simulink model "ComplexPhaseDetectorSwap"  (R2016a)
settings: Solver=VariableStepAuto  StartTime=0.0  StopTime=.05  RelTol=1e-6
PreLoadFcn:
  | Bits = 4
  | Ts=2*3/280e6
  | dBRange=11
  | maxNumErrs=500
  | maxNumBits=1e6
  | AM_Gain=AM_GainDiff;
  | AGC_Gain=AGC_GainCalc;
  | load('IIR_Coeffs.mat');
InitFcn:
  | Br= 1/(10*Ts)
  | FreqOffset=00
  | Mode=2
  | BitsPer=[2,2,1,1]
  | EbNo=50
  | N=6
undefined symbols (not defined in the file or in its folder): designMultirateFIR, DiscIntNeverNeededParam
libraries: xbsIndex_r4 x792, commfilt2 x12, commsink2 x6, dspsigops x4, commrfcorlib x2, commchan3 x2, dspfdesign x2, dspstat3 x2, dspmlti4 x1, commdigbbndpm3 x1, commrandsrc3 x1
(part 2 of 10)

== system ComplexPhaseDetectorSwap/AD9957-2 ==
  In1 : Inport
  Add3 : Sum
  Complex to Real-Imag3 : ComplexToRealImag
  FIR Interpolation : dspmlti4/FIR Interpolation  FilterSource=Auto  h=designMultirateFIR(3,1)  L=8  FilterObject=FINTERP  framing=Allow multirate processing  outputBufInitCond=0  roundingMode=Floor  overflowMode=off  firstCoeffDataTypeStr=Inherit: Same word length as input  firstCoeffMin=[]  firstCoeffMax=[]  firstCoeffLastDataTypeStr=Inherit: Same word length as input  outputDataTypeStr=Inherit: Same as accumulator  outputMin=[]  outputMax=[]  outputLastDataTypeStr=Inherit: Same as accumulator
  NCO : dspsigops/NCO  AccIncSrc=Specify via dialog  AccInc=16384*3/8  PhaseOffsetSrc=Specify via dialog  PhaseOffset=0  AccumWL=16  HasDither=off  DitherWL=4  PNgeneratorLength=19  HasPhaseQuantizer=off  TableDepth=12  HasOutputPhaseError=off  Formula=Sine and cosine  DataType=double  OutputWL=16  OutputFL=14  CompMethod=Table lookup (no interpolation)  SampleTime=Ts/8  SamplesPerFrame=1  OutputFrames=off
  PhaseDetect1 : Product
  PhaseDetect2 : Product
  Out1 : Outport
  wires:
  Add3/1 -> Out1/1
  NCO/2 -> PhaseDetect1/2
  FIR Interpolation/1 -> Complex to Real-Imag3/1
  Complex to Real-Imag3/2 -> PhaseDetect2/1
  PhaseDetect1/1 -> Add3/2
  PhaseDetect2/1 -> Add3/1
  Complex to Real-Imag3/1 -> PhaseDetect1/1
  NCO/1 -> PhaseDetect2/2
  In1/1 -> FIR Interpolation/1

== system ComplexPhaseDetectorSwap/AGCtoAWGN1 ==
  AGC : Inport
  Bias2 : Bias  Bias=100
  Gain10 : Gain  Gain=3.55
  Gain9 : Gain  Gain=-1/10
  Math Function : Math  Operator=10^u  SaturateOnIntegerOverflow=on
  Variance : Outport
  wires:
  Math Function/1 -> Gain10/1
  Gain10/1 -> Variance/1
  Gain9/1 -> Math Function/1
  Bias2/1 -> Gain9/1
  AGC/1 -> Bias2/1

== system ComplexPhaseDetectorSwap/AGCtoAWGN2 ==
  AGC : Inport
  Bias2 : Bias  Bias=100
  Gain10 : Gain  Gain=3.55
  Gain9 : Gain  Gain=-1/10
  Math Function : Math  Operator=10^u  SaturateOnIntegerOverflow=on
  Variance : Outport
  wires:
  AGC/1 -> Bias2/1
  Bias2/1 -> Gain9/1
  Gain9/1 -> Math Function/1
  Gain10/1 -> Variance/1
  Math Function/1 -> Gain10/1

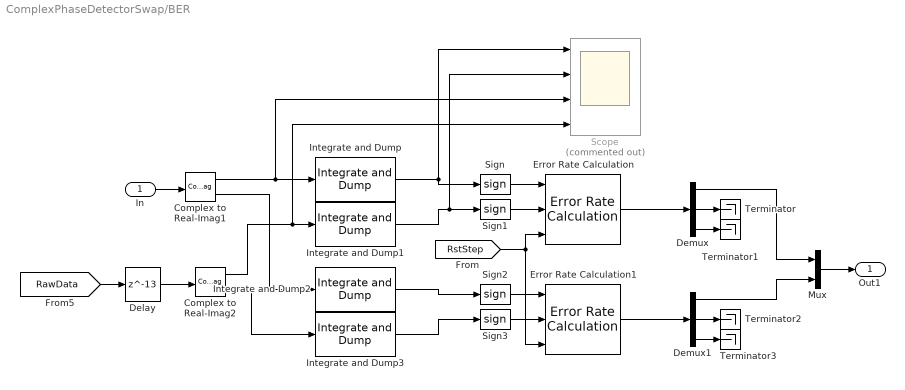
== system ComplexPhaseDetectorSwap/BER ==
  In : Inport
  Complex to Real-Imag1 : ComplexToRealImag
  Complex to Real-Imag2 : ComplexToRealImag
  Delay : Delay  DelayLength=13
  Demux : Demux  Outputs=3
  Demux1 : Demux  Outputs=3
  Error Rate Calculation : commsink2/Error Rate Calculation  N=0  st_delay=100  cp_mode=Entire frame  subframe=[]  PMode=Port  WsName=BER  RsMode2=on  stop=off  numErr=maxNumErrs  maxBits=maxNumBits
  Error Rate Calculation1 : commsink2/Error Rate Calculation  N=0  st_delay=100  cp_mode=Entire frame  subframe=[]  PMode=Port  WsName=BER  RsMode2=on  stop=off  numErr=maxNumErrs  maxBits=maxNumBits
  Integrate and Dump{,1..3} (4 alike) : commfilt2/Integrate and Dump  obssamples=1/(Br*Ts)  offsetsamples=3  nodump=off  roundingMode=Floor  overflowMode=off  outputDataTypeStr=Inherit: Same as accumulator  outputLastDataTypeStr=Inherit: Same as accumulator
  Mux : Mux  Inputs=2
  Scope : Scope  Commented=on  NumInputPorts=4
  Sign{,1..3} (4 alike) : Signum
  Terminator{,1..3} (4 alike) : Terminator
  Out1 : Outport
  wires:
  Integrate and Dump1/1 -> Scope/2, Sign1/1
  Error Rate Calculation/1 -> Demux/1
  Integrate and Dump/1 -> Scope/1, Sign/1
  Sign/1 -> Error Rate Calculation/1
  Sign1/1 -> Error Rate Calculation/2
  In/1 -> Complex to Real-Imag1/1
  Complex to Real-Imag2/1 -> Scope/4, Integrate and Dump1/1
  Delay/1 -> Complex to Real-Imag2/1
  [RawData] -> Delay/1
  Complex to Real-Imag1/1 -> Scope/3, Integrate and Dump/1
  Integrate and Dump3/1 -> Sign3/1
  Error Rate Calculation1/1 -> Demux1/1
  Integrate and Dump2/1 -> Sign2/1
  Sign2/1 -> Error Rate Calculation1/1
  Sign3/1 -> Error Rate Calculation1/2
  Complex to Real-Imag2/2 -> Integrate and Dump3/1
  [RstStep] -> Error Rate Calculation1/3, Error Rate Calculation/3
  Complex to Real-Imag1/2 -> Integrate and Dump2/1
  Demux/1 -> Mux/1
  Demux1/1 -> Mux/2
  Demux/2 -> Terminator/1
  Demux/3 -> Terminator1/1
  Demux1/2 -> Terminator2/1
  Demux1/3 -> Terminator3/1
  Mux/1 -> Out1/1

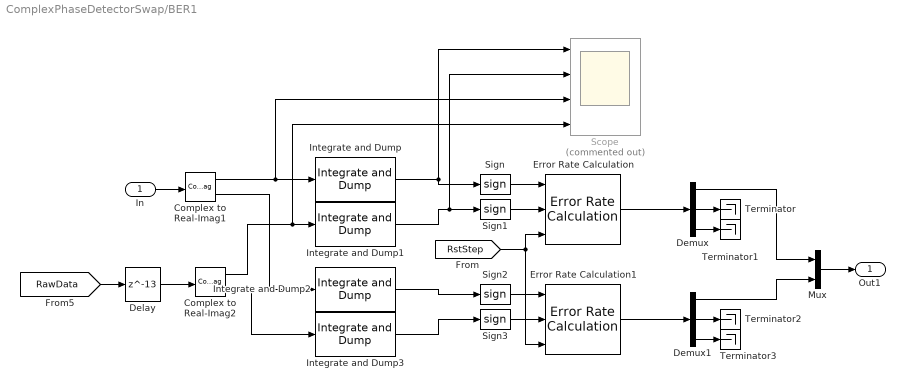
== system ComplexPhaseDetectorSwap/BER1 ==
  In : Inport
  Complex to Real-Imag1 : ComplexToRealImag
  Complex to Real-Imag2 : ComplexToRealImag
  Delay : Delay  DelayLength=13
  Demux : Demux  Outputs=3
  Demux1 : Demux  Outputs=3
  Error Rate Calculation : commsink2/Error Rate Calculation  N=0  st_delay=100  cp_mode=Entire frame  subframe=[]  PMode=Port  WsName=BER  RsMode2=on  stop=off  numErr=maxNumErrs  maxBits=maxNumBits
  Error Rate Calculation1 : commsink2/Error Rate Calculation  N=0  st_delay=100  cp_mode=Entire frame  subframe=[]  PMode=Port  WsName=BER  RsMode2=on  stop=off  numErr=maxNumErrs  maxBits=maxNumBits
  Integrate and Dump{,1..3} (4 alike) : commfilt2/Integrate and Dump  obssamples=1/(Br*Ts)  offsetsamples=3  nodump=off  roundingMode=Floor  overflowMode=off  outputDataTypeStr=Inherit: Same as accumulator  outputLastDataTypeStr=Inherit: Same as accumulator
  Mux : Mux  Inputs=2
  Scope : Scope  Commented=on  NumInputPorts=4
  Sign{,1..3} (4 alike) : Signum
  Terminator{,1..3} (4 alike) : Terminator
  Out1 : Outport
  wires:
  Mux/1 -> Out1/1
  Demux1/3 -> Terminator3/1
  Demux1/2 -> Terminator2/1
  Demux/3 -> Terminator1/1
  Demux/2 -> Terminator/1
  Demux1/1 -> Mux/2
  Demux/1 -> Mux/1
  Complex to Real-Imag1/2 -> Integrate and Dump2/1
  [RstStep] -> Error Rate Calculation/3, Error Rate Calculation1/3
  Complex to Real-Imag2/2 -> Integrate and Dump3/1
  Sign3/1 -> Error Rate Calculation1/2
  Sign2/1 -> Error Rate Calculation1/1
  Integrate and Dump2/1 -> Sign2/1
  Error Rate Calculation1/1 -> Demux1/1
  Integrate and Dump3/1 -> Sign3/1
  Complex to Real-Imag1/1 -> Integrate and Dump/1, Scope/3
  [RawData] -> Delay/1
  Delay/1 -> Complex to Real-Imag2/1
  Complex to Real-Imag2/1 -> Integrate and Dump1/1, Scope/4
  In/1 -> Complex to Real-Imag1/1
  Sign1/1 -> Error Rate Calculation/2
  Sign/1 -> Error Rate Calculation/1
  Integrate and Dump/1 -> Sign/1, Scope/1
  Error Rate Calculation/1 -> Demux/1
  Integrate and Dump1/1 -> Sign1/1, Scope/2

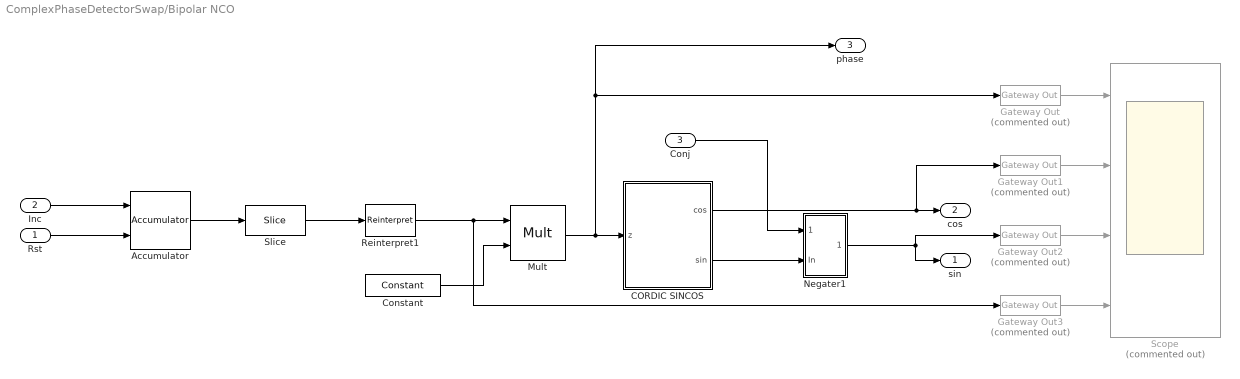
== system ComplexPhaseDetectorSwap/Bipolar NCO ==
  Rst : Inport
  Inc : Inport  Port=2
  Conj : Inport  Port=3
  Accumulator : xbsIndex_r4/Accumulator  operation=Add  n_bits=18+Bits  overflow=Wrap  scale=1  rst=on  hasbypass=off  infoeditControl=reset for floating point data type must be asserted for a minimum of 2 cycles  en=off  latency=1  msb_inp=100  msb=100  lsb=-100  use_behavioral_HDL=on  implementation=Fabric  dbl_ovrd=off  block_type=accum
  CORDIC SINCOS : Subsystem  mask(Xilinx CORDIC SINCOS){stages=17, pe_nbits=21, pe_binpt=17, pipeline_x=ones(1,17), prev_stages=17, pipeline=[1  1  1  1  1  1  1  1  1  1  1  1  1  1  1  1  1]}
      mask prompts: stages "Number of Processing Elements (integer value starting from 1)"; pe_nbits "Input Data Width"; pe_binpt "Input Binary Point Position"; pipeline_x "Latency for each Processing Element [1 0 0 1]"; prev_stages "Previous Number of Stages"; pipeline "Previous Pipeline Values"
      mask help: A parallel implementation, circular rotation mode CORDIC processor for calculating Sine and Cosine of input angle z. The number of iteration stages (and resultant output accuracy) and the processor arithmetic precision are controlled by the mask customization.
      mask init:
      | [bg,fg] = xlcmap('XBlock',0);
      | iPos = get_param(gcb,'Position');
      | iWidth=iPos(3)-iPos(1); iHeight=iPos(4)-iPos(2);
      | iCx=iWidth/2;
      | iCy=iHeight/2;
      | [logoX, logoY] = xlogo(iPos);
      | sav_gcb=gcb;
      | stages = round(sum(abs(stages)));
      | if (stages == 0)
      | 	stages = prev_stages;
      | end
      | x = zeros(1,stages);
      | pipe_size = max(size(pipeline_x));
      | if pipe_size >= stages
      | 	x(1,1:stages) = pipeline_x(1,1:stages);
      | else
      | 	x(1,1:pipe_size) = pipeline_x(1,1:pipe_size);
      | end
      | 
      | if (stages ~=prev_stages)
      | 	pipeline=x;
      | 	cordic_pe = find_system(gcb, 'lookUnderMasks', 'all', 'FollowLinks','on','masktype', 'CORDIC parallel PE');
      |     
      |   a=find_system(cordic_pe{1}, 'lookUnderMasks', 'all', 'FollowLinks','on','masktype', 'CORDIC iteration PE');
      |   for i= 2:length(a)
      |     for j=1:3
      | 	  delete_line(cordic_pe{1}, ['CORDIC PE' int2str(i-1) '/' int2str(j)], ['CORDIC PE' int2str(i) '/' int2str(j)]);
      |     end
      |   end
      |     if length(a)>0,
      |       delete_line(cordic_pe{1}, 'x/1', 'CORDIC PE1/1');
      |       delete_line(cordic_pe{1}, 'y/1', 'CORDIC PE1/2');
      |       delete_line(cordic_pe{1}, 'z/1', 'CORDIC PE1/3');
      |       delete_line(cordic_pe{1}, ['CORDIC PE' int2str(length(a)) '/1'],'X/1');
      |       delete_line(cordic_pe{1}, ['CORDIC PE' int2str(length(a)) '/2'],'Y/1');
      |       delete_line(cordic_pe{1}, ['CORDIC PE' int2str(length(a)) '/3'],'Terminator/1');
      |     elseif length(a)==0
      |       temp_port=get_param([cordic_pe{1} '/x'],'porthandles');
      |       temp_line=get_param(temp_port.Outport,'line');
      |       if temp_line>=0  delete_line(temp_line); end
      |       temp_port=get_param([cordic_pe{1} '/y'],'porthandles');
      |       temp_line=get_param(temp_port.Outport,'line');
      |       if temp_line>=0  delete_line(temp_line); end
      |       temp_port=get_param([cordic_pe{1} '/z'],'porthandles');
      |       temp_line=get_param(temp_port.Outport,'line');
      |       if temp_line>=0  delete_line(temp_line); end
      |     end
      | 
      |     for i=2:length(a)
      |       delete_block(a{i});
      |     end
      |     for i=2:stages,
      |         add_block([cordic_pe{1} '/CORDIC PE1'], [cordic_pe{1} '/CORDIC PE' int2str(i)], 'ii', int2str(i-1),'pe_nbits', 'pe_nbits','pe_binpt', 'pe_binpt','pipeline',['pipeline(1,' int2str(i) ')'],'position',[150+(i-1)*125, 70, 205+(i-1)*125, 130]);
      |     end
      | 
      |     for i= 2:stages,
      |       for j=1:3
      | 		add_line(cordic_pe{1}, ['CORDIC PE' int2str(i-1) '/' int2str(j)], ['CORDIC PE' int2str(i) '/' int2str(j)], 'autorouting', 'on');
      |       end
      |     end
      | 
      |     if stages==0
      |       add_line(cordic_pe{1}, 'x/1', 'X/1', 'autorouting', 'on');
      |       add_line(cordic_pe{1}, 'y/1', 'Terminator/1', 'autorouting', 'on');
      |       add_line(cordic_pe{1}, 'z/1', 'Z/1', 'autorouting', 'on');
      |     elseif stages>0
      |       add_line(cordic_pe{1}, 'x/1', 'CORDIC PE1/1', 'autorouting', 'on');
      |       add_line(cordic_pe{1}, 'y/1', 'CORDIC PE1/2', 'autorouting', 'on');
      |       add_line(cordic_pe{1}, 'z/1', 'CORDIC PE1/3', 'autorouting', 'on');
      | 
      |       set_param([cordic_pe{1} '/' 'X'], 'Position', [150+stages*125, 72, 180+stages*125, 86]);
      |       set_param([cordic_pe{1} '/' 'Y'], 'Position', [210+stages*125, 92, 225+stages*125, 108]);
      |       set_param([cordic_pe{1} '/' 'Terminator'], 'Position', [240+stages*125, 113, 270+stages*125, 127]);
      | 
      |       add_line(cordic_pe{1}, ['CORDIC PE' int2str(stages) '/1'], 'X/1', 'autorouting', 'on');
      |       add_line(cordic_pe{1}, ['CORDIC PE' int2str(stages) '/2'], 'Y/1', 'autorouting', 'on');
      |       add_line(cordic_pe{1}, ['CORDIC PE' int2str(stages) '/3'],'Terminator/1', 'autorouting', 'on');
      | 
      |       % force a "compile" of the constituent constant blocks to
      |       % workaround a data propagation problem
      |       find_system(cordic_pe{1}, 'lookUnderMasks', 'all', 'FollowLinks', 'on', 'MaskType','Xilinx Constant Block');
      |   end
      | 	set_param(sav_gcb, 'prev_stages', int2str(stages));
      | 	set_param(sav_gcb, 'pipeline', [ '[' int2str(x) ']']);
      | else
      | 	if (sum(pipeline~=x))
      | 		set_param(gcb, 'pipeline', [ '[' int2str(x) ']']);
      | 	end
      | end
      | str = sprintf('-%d',sum(x) + 3);
      settings: CopyFcn=set_param(gcb, 'MaskSelfModifiable', 'on', 'LinkStatus', 'none');
      mask Help: eval('');xlDoc('-book','sysgen','-topic','CORDIC_SINCOS');
      mask Display:
      | patch([0 iWidth iWidth 0],[0 0 iHeight iHeight] , bg);
      | patch(logoX,logoY , fg);
      | text(iCx-6,iCy,'z');
      | text(iCx,iCy+4,str);
      | port_label('input',1,'z');
      | port_label('output',1,'cos');
      | port_label('output',2,'sin');
      | plot([0 0 iWidth iWidth 0], [0 iHeight iHeight 0 0]);
  Constant : xbsIndex_r4/Constant  const=pi()  gui_display_data_type=Fixed-point  arith_type=Signed (2's comp)  n_bits=18  bin_pt=14  preci_type=Single  exp_width=8  frac_width=24  explicit_period=off  period=1  equ=P=C  opselect=C  inp2=PCIN>>17  opr=+  inp1=P  carry=CIN  dbl_ovrd=off  block_type=constant
  Gateway Out{,1..3} (4 alike) : xbsIndex_r4/Gateway Out  Commented=on  inherit_from_input=off  hdl_port=on  rows=1  columns=1  UseAsDAC=off  DACChannel='1'  interface=None  automatic_assignment=on  address_offset=hex2dec('00')  intf_name=''  intf_description=''  timing_constraint=None  locs_specified=off  LOCs={}  io_standard={}  block_type=gatewayout
  Mult : xbsIndex_r4/Mult  precision=User Defined  arith_type="Signed  (2's comp)"  n_bits=21  bin_pt=17  quantization=Truncate  overflow=Saturate  en=off  latency=3  use_behavioral_HDL=off  opt=Speed  use_embedded=on  optimum_pipeline=off  pipeline=on  dbl_ovrd=off  use_rpm=on  placement_style=Triangular  block_type=mult
  Negater1 : Subsystem
  Reinterpret1 : xbsIndex_r4/Reinterpret  force_arith_type=on  arith_type="Signed  (2's comp)"  force_bin_pt=on  bin_pt=17  block_type=reinterpret
  Scope : Scope  Commented=on  NumInputPorts=4
  Slice : xbsIndex_r4/Slice  nbits=18  boolean_output=off  mode=Upper Bit Location + Width  bit1=0  base1=MSB of Input  bit0=0  base0=LSB of Input  dbl_ovrd=off  block_type=slice
  sin : Outport
  cos : Outport  Port=2
  phase : Outport  Port=3
  wires:
  CORDIC SINCOS/1(cos) -> Gateway Out1/1, cos/1
  Negater1/1(Out) -> sin/1, Gateway Out2/1
  Gateway Out2/1 -> Scope/3
  Gateway Out/1 -> Scope/1
  Gateway Out1/1 -> Scope/2
  Accumulator/1 -> Slice/1
  Constant/1 -> Mult/2
  Gateway Out3/1 -> Scope/4
  Inc/1 -> Accumulator/1
  Slice/1 -> Reinterpret1/1
  Reinterpret1/1 -> Gateway Out3/1, Mult/1
  Rst/1 -> Accumulator/2
  CORDIC SINCOS/2(sin) -> Negater1/2(In)
  Conj/1 -> Negater1/1(Neg)
  Mult/1 -> phase/1, Gateway Out/1, CORDIC SINCOS/1(z)

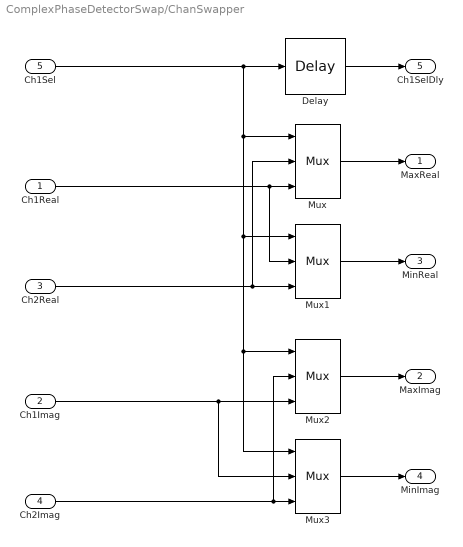
== system ComplexPhaseDetectorSwap/ChanSwapper ==
  Ch1Real : Inport
  Ch1Imag : Inport  Port=2
  Ch2Real : Inport  Port=3
  Ch2Imag : Inport  Port=4
  Ch1Sel : Inport  Port=5
  Delay : xbsIndex_r4/Delay  rst=off  infoeditControl=Selection of Reset will increase slice count due to use of real FFs and instead of SRLs  en=off  latency=1  reg_retiming=off  dbl_ovrd=off  block_type=delay
  Mux{,1..3} (4 alike) : xbsIndex_r4/Mux  inputs=2  en=off  latency=1  precision=Full  arith_type=Unsigned  n_bits=16  bin_pt=14  quantization=Truncate  overflow=Wrap  dbl_ovrd=off  block_type=mux
  MaxReal : Outport
  MaxImag : Outport  Port=2
  "MinReal " : Outport  Port=3
  MinImag : Outport  Port=4
  Ch1SelDly : Outport  Port=5
  wires:
  Ch1Sel/1 -> Mux3/1, Mux2/1, Mux1/1, Mux/1, Delay/1
  Ch2Imag/1 -> Mux2/2, Mux3/3
  Ch2Real/1 -> Mux1/3, Mux/2
  Ch1Real/1 -> Mux1/2, Mux/3
  Ch1Imag/1 -> Mux3/2, Mux2/3
  Mux/1 -> MaxReal/1
  Mux1/1 -> "MinReal "/1
  Mux2/1 -> MaxImag/1
  Mux3/1 -> MinImag/1
  Delay/1 -> Ch1SelDly/1

== system ComplexPhaseDetectorSwap/Conjugate ==
  In1 : Inport
  Complex to Real-Imag : ComplexToRealImag
  Real-Imag to Complex : RealImagToComplex
  Unary Minus : UnaryMinus
  Out1 : Outport
  wires:
  In1/1 -> Complex to Real-Imag/1
  Complex to Real-Imag/1 -> Real-Imag to Complex/1
  Complex to Real-Imag/2 -> Unary Minus/1
  Unary Minus/1 -> Real-Imag to Complex/2
  Real-Imag to Complex/1 -> Out1/1

== system ComplexPhaseDetectorSwap/Cordic ATan ==
  note: If Real=Imag=0, the Cordic goes to 180°, not 0.
  Imag : Inport
  Real : Inport  Port=2
  CORDIC ATAN : Subsystem  mask(Xilinx CORDIC ATAN){stages=10, pe_nbits=18, pe_binpt=15, pipeline_x=ones(1,10), prev_stages=10, pipeline=[1  1  1  1  1  1  1  1  1  1]}
      mask prompts: stages "Number of Processing Elements (integer value starting from 1)"; pe_nbits "X, Y Data Width"; pe_binpt "X, Y Binary Point Position"; pipeline_x "Latency for each Processing Element [1 0 0 1]"; prev_stages "Previous Number of Stages"; pipeline "Previous Pipeline Values"
      mask help: A parallel implementation, circular vectoring mode CORDIC processor for performing rectangular-to-polar conversion. The number of iteration stages (and resultant output accuracy) and the processor arithmetic precision are controlled by the mask customization.
      mask init:
      | [bg,fg] = xlcmap('XBlock',0);
      | iPos = get_param(gcb,'Position');
      | iWidth=iPos(3)-iPos(1); iHeight=iPos(4)-iPos(2);
      | iCx=iWidth/2;
      | iCy=iHeight/2;
      | [logoX, logoY] = xlogo(iPos);
      | sav_gcb=gcb;
      | stages = round(sum(abs(stages)));
      | if (stages == 0)
      | 	stages = prev_stages;
      | end
      | x = zeros(1,stages);
      | pipe_size = max(size(pipeline_x));
      | if pipe_size >= stages
      | 	x(1,1:stages) = pipeline_x(1,1:stages);
      | else
      | 	x(1,1:pipe_size) = pipeline_x(1,1:pipe_size);
      | end
      | 
      | if (stages ~=prev_stages)
      | 	pipeline=x;
      | 	cordic_pe = find_system(gcb, 'lookUnderMasks', 'all', 'FollowLinks','on','masktype', 'CORDIC parallel PE');
      |     
      |   a=find_system(cordic_pe{1}, 'lookUnderMasks', 'all', 'FollowLinks','on','masktype', 'CORDIC iteration PE');
      |   for i= 2:length(a)
      |     for j=1:3
      | 	  delete_line(cordic_pe{1}, ['CORDIC PE' int2str(i-1) '/' int2str(j)], ['CORDIC PE' int2str(i) '/' int2str(j)]);
      |     end
      |   end
      |     if length(a)>0,
      |       delete_line(cordic_pe{1}, 'x/1', 'CORDIC PE1/1');
      |       delete_line(cordic_pe{1}, 'y/1', 'CORDIC PE1/2');
      |       delete_line(cordic_pe{1}, 'z/1', 'CORDIC PE1/3');
      |       delete_line(cordic_pe{1}, ['CORDIC PE' int2str(length(a)) '/1'],'X/1');
      |       delete_line(cordic_pe{1}, ['CORDIC PE' int2str(length(a)) '/2'],'Terminator/1');
      |       delete_line(cordic_pe{1}, ['CORDIC PE' int2str(length(a)) '/3'],'Z/1');
      |     elseif length(a)==0
      |       temp_port=get_param([cordic_pe{1} '/x'],'porthandles');
      |       temp_line=get_param(temp_port.Outport,'line');
      |       if temp_line>=0  delete_line(temp_line); end
      |       temp_port=get_param([cordic_pe{1} '/y'],'porthandles');
      |       temp_line=get_param(temp_port.Outport,'line');
      |       if temp_line>=0  delete_line(temp_line); end
      |       temp_port=get_param([cordic_pe{1} '/z'],'porthandles');
      |       temp_line=get_param(temp_port.Outport,'line');
      |       if temp_line>=0  delete_line(temp_line); end
      |     end
      | 
      |     for i=2:length(a)
      |       delete_block(a{i});
      |     end
      |     for i=2:stages,
      |         add_block([cordic_pe{1} '/CORDIC PE1'], [cordic_pe{1} '/CORDIC PE' int2str(i)], 'ii', int2str(i-1),'pe_nbits', 'pe_nbits','pe_binpt', 'pe_binpt','pipeline',['pipeline(1,' int2str(i) ')'],'position',[150+(i-1)*125, 70, 205+(i-1)*125, 130]);
      |     end
      | 
      |     for i= 2:stages,
      |       for j=1:3
      | 		add_line(cordic_pe{1}, ['CORDIC PE' int2str(i-1) '/' int2str(j)], ['CORDIC PE' int2str(i) '/' int2str(j)], 'autorouting', 'on');
      |       end
      |     end
      | 
      |     if stages==0
      |       add_line(cordic_pe{1}, 'x/1', 'X/1', 'autorouting', 'on');
      |       add_line(cordic_pe{1}, 'y/1', 'Terminator/1', 'autorouting', 'on');
      |       add_line(cordic_pe{1}, 'z/1', 'Z/1', 'autorouting', 'on');
      |     elseif stages>0
      |       add_line(cordic_pe{1}, 'x/1', 'CORDIC PE1/1', 'autorouting', 'on');
      |       add_line(cordic_pe{1}, 'y/1', 'CORDIC PE1/2', 'autorouting', 'on');
      |       add_line(cordic_pe{1}, 'z/1', 'CORDIC PE1/3', 'autorouting', 'on');
      | 
      |       set_param([cordic_pe{1} '/' 'X'], 'Position', [150+stages*125, 72, 180+stages*125, 86]);
      |       set_param([cordic_pe{1} '/' 'Terminator'], 'Position', [210+stages*125, 92, 225+stages*125, 108]);
      |       set_param([cordic_pe{1} '/' 'Z'], 'Position', [240+stages*125, 113, 270+stages*125, 127]);
      | 
      |       add_line(cordic_pe{1}, ['CORDIC PE' int2str(stages) '/1'], 'X/1', 'autorouting', 'on');
      |       add_line(cordic_pe{1}, ['CORDIC PE' int2str(stages) '/2'], 'Terminator/1', 'autorouting', 'on');
      |       add_line(cordic_pe{1}, ['CORDIC PE' int2str(stages) '/3'],'Z/1', 'autorouting', 'on');
      | 
      |       % force a "compile" of the constituent constant blocks to
      |       % workaround a data propagation problem
      |       find_system(cordic_pe{1}, 'lookUnderMasks', 'all', 'FollowLinks', 'on', 'MaskType','Xilinx Constant Block');
      |   end
      | 	set_param(sav_gcb, 'prev_stages', int2str(stages));
      | 	set_param(sav_gcb, 'pipeline', [ '[' int2str(x) ']']);
      | else
      | 	if (sum(pipeline~=x))
      | 		set_param(gcb, 'pipeline', [ '[' int2str(x) ']']);
      | 	end
      | end
      | str = sprintf('-%d',sum(x) + 3);
      settings: CopyFcn=set_param(gcb, 'MaskSelfModifiable', 'on', 'LinkStatus', 'none');
      mask Help: eval('');xlDoc('-book','sysgen','-topic','CORDIC_ATAN');
      mask Display:
      | patch([0 iWidth iWidth 0],[0 0 iHeight iHeight] , bg);
      | patch(logoX,logoY , fg);
      | text(iCx-6,iCy,'z');
      | text(iCx,iCy+4,str);
      | port_label('input',1,'x');
      | port_label('input',2,'y');
      | port_label('output',1,'mag');
      | port_label('output',2,'atan');
      | plot([0 0 iWidth iWidth 0], [0 iHeight iHeight 0 0]);
  Constant : xbsIndex_r4/Constant  const=0  gui_display_data_type=Fixed-point  arith_type=Signed (2's comp)  n_bits=18  bin_pt=15  preci_type=Single  exp_width=8  frac_width=24  explicit_period=off  period=1  equ=P=C  opselect=C  inp2=PCIN>>17  opr=+  inp1=P  carry=CIN  dbl_ovrd=off  block_type=constant
  Mux : xbsIndex_r4/Mux  inputs=2  en=off  latency=1  precision=Full  arith_type=Unsigned  n_bits=16  bin_pt=14  quantization=Truncate  overflow=Wrap  dbl_ovrd=off  block_type=mux
  Relational1 : xbsIndex_r4/Relational  mode=a>b  op_type=Bool  en=off  latency=0  dbl_ovrd=off  block_type=relational
  Phase : Outport
  wires:
  Real/1 -> CORDIC ATAN/1(x)
  Imag/1 -> CORDIC ATAN/2(y)
  CORDIC ATAN/1(X) -> Relational1/1
  Mux/1 -> Phase/1
  CORDIC ATAN/2(Z) -> Mux/3
  Constant/1 -> Mux/2, Relational1/2
  Relational1/1 -> Mux/1

== system ComplexPhaseDetectorSwap/Knob ==

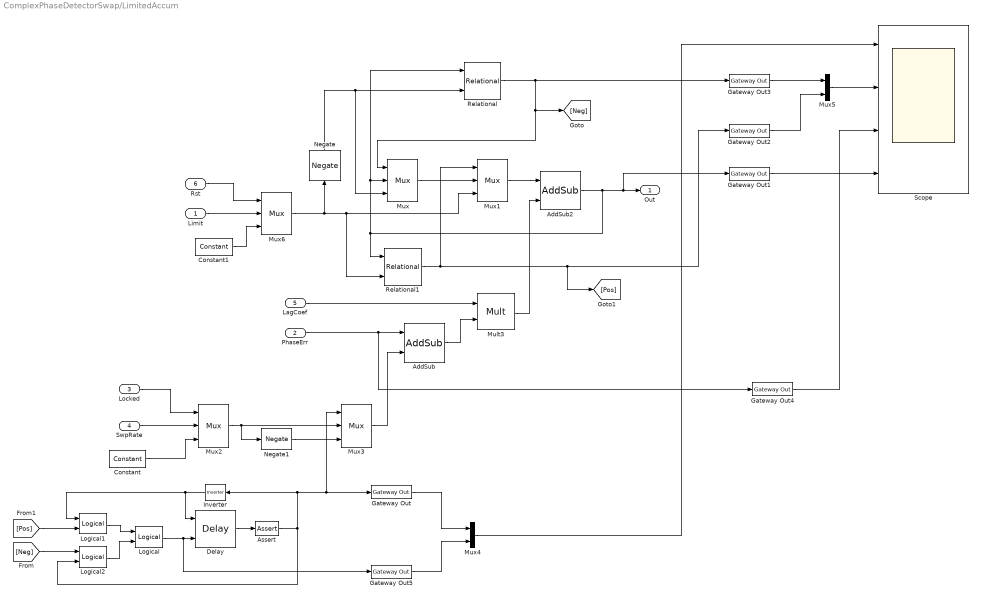
== system ComplexPhaseDetectorSwap/LimitedAccum ==
  Limit : Inport
  PhaseErr : Inport  Port=2
  Locked : Inport  Port=3
  SwpRate : Inport  Port=4
  LagCoef : Inport  Port=5
  Rst : Inport  Port=6
  AddSub : xbsIndex_r4/AddSub  mode=Addition  use_carryin=off  use_carryout=off  en=off  latency=1  precision=Full  arith_type=Unsigned  n_bits=16  bin_pt=14  quantization=Truncate  overflow=Wrap  use_behavioral_HDL=off  hw_selection=Fabric  pipelined=off  dbl_ovrd=off  block_type=addsub
  AddSub2 : xbsIndex_r4/AddSub  mode=Addition  use_carryin=off  use_carryout=off  en=off  latency=1  precision=User Defined  arith_type="Signed  (2's comp)"  n_bits=32  bin_pt=17  quantization="Round  (unbiased: +/- Inf)"  overflow=Wrap  use_behavioral_HDL=off  hw_selection=Fabric  pipelined=off  dbl_ovrd=off  block_type=addsub
  Assert : xbsIndex_r4/Assert  assert_type=on  type_source=Explicitly  gui_display_data_type=Boolean  arith_type=Boolean  n_bits=1  bin_pt=14  preci_type=Single  exp_width=8  frac_width=24  assert_rate=off  rate_source=Explicitly  period=1  output_port=on  block_type=assert
  Constant : xbsIndex_r4/Constant  const=0  gui_display_data_type=Fixed-point  arith_type=Unsigned  n_bits=8  bin_pt=5  preci_type=Single  exp_width=8  frac_width=24  explicit_period=on  period=Ts  equ=P=C  opselect=C  inp2=PCIN>>17  opr=+  inp1=P  carry=CIN  dbl_ovrd=off  block_type=constant
  Constant1 : xbsIndex_r4/Constant  const=0  gui_display_data_type=Fixed-point  arith_type=Unsigned  n_bits=14  bin_pt=0  preci_type=Single  exp_width=8  frac_width=24  explicit_period=on  period=Ts  equ=P=C  opselect=C  inp2=PCIN>>17  opr=+  inp1=P  carry=CIN  dbl_ovrd=off  block_type=constant
  Delay : xbsIndex_r4/Delay  rst=off  infoeditControl=Selection of Reset will increase slice count due to use of real FFs and instead of SRLs  en=on  latency=1  reg_retiming=off  dbl_ovrd=off  block_type=delay
  Gateway Out{,1..5} (6 alike) : xbsIndex_r4/Gateway Out  inherit_from_input=off  hdl_port=off  rows=1  columns=1  UseAsDAC=off  DACChannel='1'  interface=None  automatic_assignment=on  address_offset=hex2dec('00')  intf_name=''  intf_description=''  timing_constraint=None  locs_specified=off  LOCs={}  io_standard={}  block_type=gatewayout
  Inverter : xbsIndex_r4/Inverter  en=off  latency=0  dbl_ovrd=off  block_type=inv
  Logical : xbsIndex_r4/Logical  logical_function=OR  inputs=2  en=off  latency=0  precision=Full  arith_type=Unsigned  n_bits=16  bin_pt=0  align_bp=on  dbl_ovrd=off  block_type=logical
  Logical1 : xbsIndex_r4/Logical  logical_function=AND  inputs=2  en=off  latency=0  precision=Full  arith_type=Unsigned  n_bits=16  bin_pt=0  align_bp=on  dbl_ovrd=off  block_type=logical
  Logical2 : xbsIndex_r4/Logical  logical_function=AND  inputs=2  en=off  latency=0  precision=Full  arith_type=Unsigned  n_bits=16  bin_pt=0  align_bp=on  dbl_ovrd=off  block_type=logical
  Mult3 : xbsIndex_r4/Mult  precision=User Defined  arith_type="Signed  (2's comp)"  n_bits=18+Bits  bin_pt=17  quantization="Round  (unbiased: +/- Inf)"  overflow=Wrap  en=off  latency=3  use_behavioral_HDL=off  opt=Speed  use_embedded=on  optimum_pipeline=off  pipeline=on  dbl_ovrd=off  use_rpm=on  placement_style=Triangular  block_type=mult
  Mux{,1..2,6} (4 alike) : xbsIndex_r4/Mux  inputs=2  en=off  latency=0  precision=Full  arith_type=Unsigned  n_bits=16  bin_pt=14  quantization=Truncate  overflow=Wrap  dbl_ovrd=off  block_type=mux
  Mux3 : xbsIndex_r4/Mux  inputs=2  en=off  latency=1  precision=Full  arith_type=Unsigned  n_bits=16  bin_pt=14  quantization=Truncate  overflow=Wrap  dbl_ovrd=off  block_type=mux
  Mux4 : Mux  Inputs=2
  Mux5 : Mux  Inputs=2
  Negate : xbsIndex_r4/Negate  precision=Full  arith_type=Unsigned  n_bits=Bits+18  bin_pt=14  quantization=Truncate  overflow=Wrap  en=off  latency=0  dbl_ovrd=off  block_type=negate
  Negate1 : xbsIndex_r4/Negate  precision=Full  arith_type=Unsigned  n_bits=Bits+18  bin_pt=14  quantization=Truncate  overflow=Wrap  en=off  latency=0  dbl_ovrd=off  block_type=negate
  Relational : xbsIndex_r4/Relational  mode=a<b  op_type=Bool  en=off  latency=0  dbl_ovrd=off  block_type=relational
  Relational1 : xbsIndex_r4/Relational  mode=a>b  op_type=Bool  en=off  latency=0  dbl_ovrd=off  block_type=relational
  Scope : Scope  NumInputPorts=4
  Out : Outport
  wires:
  Mult3/1 -> AddSub2/2
  AddSub2/1 -> Relational/1, Mux/2, Relational1/1, Out/1, Gateway Out1/1
  Mux/1 -> Mux1/2
  Mux6/1 -> Negate/1, Mux1/3, Relational1/2
  Relational/1 -> [Neg], Mux/1, Gateway Out3/1
  Relational1/1 -> Mux1/1, [Pos], Gateway Out2/1
  Gateway Out1/1 -> Scope/4
  Gateway Out3/1 -> Mux5/1
  Mux4/1 -> Scope/1
  Gateway Out2/1 -> Mux5/2
  Mux1/1 -> AddSub2/1
  Negate/1 -> Relational/2, Mux/3
  PhaseErr/1 -> Gateway Out4/1, AddSub/1
  LagCoef/1 -> Mult3/1
  AddSub/1 -> Mult3/2
  Locked/1 -> Mux2/1
  Constant/1 -> Mux2/3
  Mux2/1 -> Negate1/1, Mux3/2
  SwpRate/1 -> Mux2/2
  Negate1/1 -> Mux3/3
  Mux3/1 -> AddSub/2
  Delay/1 -> Assert/1
  [Pos] -> Logical1/2
  [Neg] -> Logical2/1
  Logical/1 -> Gateway Out5/1, Delay/2
  Inverter/1 -> Delay/1, Logical1/1
  Assert/1 -> Logical2/2, Gateway Out/1, Mux3/1, Inverter/1
  Logical1/1 -> Logical/1
  Logical2/1 -> Logical/2
  Mux5/1 -> Scope/2
  Gateway Out4/1 -> Scope/3
  Gateway Out/1 -> Mux4/1
  Gateway Out5/1 -> Mux4/2
  Limit/1 -> Mux6/2
  Rst/1 -> Mux6/1
  Constant1/1 -> Mux6/3

== system ComplexPhaseDetectorSwap/LockImag ==
  In : Inport
  Sub : Inport  Port=2
  Rst_n : Inport  Port=3
  Constant : xbsIndex_r4/Constant  const=0  gui_display_data_type=Fixed-point  arith_type=Unsigned  n_bits=13  bin_pt=0  preci_type=Single  exp_width=8  frac_width=24  explicit_period=off  period=1  equ=P=C  opselect=C  inp2=PCIN>>17  opr=+  inp1=P  carry=CIN  dbl_ovrd=off  block_type=constant
  LockReal : xbsIndex_r4/AddSub  mode=Addition or Subtraction  use_carryin=off  use_carryout=off  en=off  latency=1  precision=User Defined  arith_type=Unsigned  n_bits=13  bin_pt=0  quantization=Truncate  overflow=Saturate  use_behavioral_HDL=off  hw_selection=Fabric  pipelined=off  dbl_ovrd=off  block_type=addsub
  Mux : xbsIndex_r4/Mux  inputs=2  en=off  latency=0  precision=Full  arith_type=Unsigned  n_bits=16  bin_pt=14  quantization=Truncate  overflow=Wrap  dbl_ovrd=off  block_type=mux
  Out : Outport
  wires:
  Rst_n/1 -> Mux/1
  Constant/1 -> Mux/2
  Mux/1 -> LockReal/1
  LockReal/1 -> Out/1, Mux/3
  Sub/1 -> LockReal/3
  In/1 -> LockReal/2

== system ComplexPhaseDetectorSwap/LockReal ==
  In : Inport
  Sub : Inport  Port=2
  Rst_n : Inport  Port=3
  Constant : xbsIndex_r4/Constant  const=0  gui_display_data_type=Fixed-point  arith_type=Unsigned  n_bits=13  bin_pt=0  preci_type=Single  exp_width=8  frac_width=24  explicit_period=off  period=1  equ=P=C  opselect=C  inp2=PCIN>>17  opr=+  inp1=P  carry=CIN  dbl_ovrd=off  block_type=constant
  LockReal : xbsIndex_r4/AddSub  mode=Addition or Subtraction  use_carryin=off  use_carryout=off  en=off  latency=1  precision=User Defined  arith_type=Unsigned  n_bits=13  bin_pt=0  quantization=Truncate  overflow=Saturate  use_behavioral_HDL=off  hw_selection=Fabric  pipelined=off  dbl_ovrd=off  block_type=addsub
  Mux : xbsIndex_r4/Mux  inputs=2  en=off  latency=0  precision=Full  arith_type=Unsigned  n_bits=16  bin_pt=14  quantization=Truncate  overflow=Wrap  dbl_ovrd=off  block_type=mux
  Out : Outport
  wires:
  In/1 -> LockReal/2
  Sub/1 -> LockReal/3
  LockReal/1 -> Mux/3, Out/1
  Mux/1 -> LockReal/1
  Constant/1 -> Mux/2
  Rst_n/1 -> Mux/1

== system ComplexPhaseDetectorSwap/Negater2 ==
  Neg : Inport
  In : Inport  Port=2
  Mux11 : xbsIndex_r4/Mux  inputs=2  en=off  latency=1  precision=Full  arith_type=Unsigned  n_bits=16  bin_pt=14  quantization=Truncate  overflow=Wrap  dbl_ovrd=off  block_type=mux
  Negate1 : xbsIndex_r4/Negate  precision=User Defined  arith_type="Signed  (2's comp)"  n_bits=18  bin_pt=15  quantization=Truncate  overflow=Saturate  en=off  latency=0  dbl_ovrd=off  block_type=negate
  Out : Outport
  wires:
  Neg/1 -> Mux11/1
  In/1 -> Negate1/1, Mux11/2
  Mux11/1 -> Out/1
  Negate1/1 -> Mux11/3

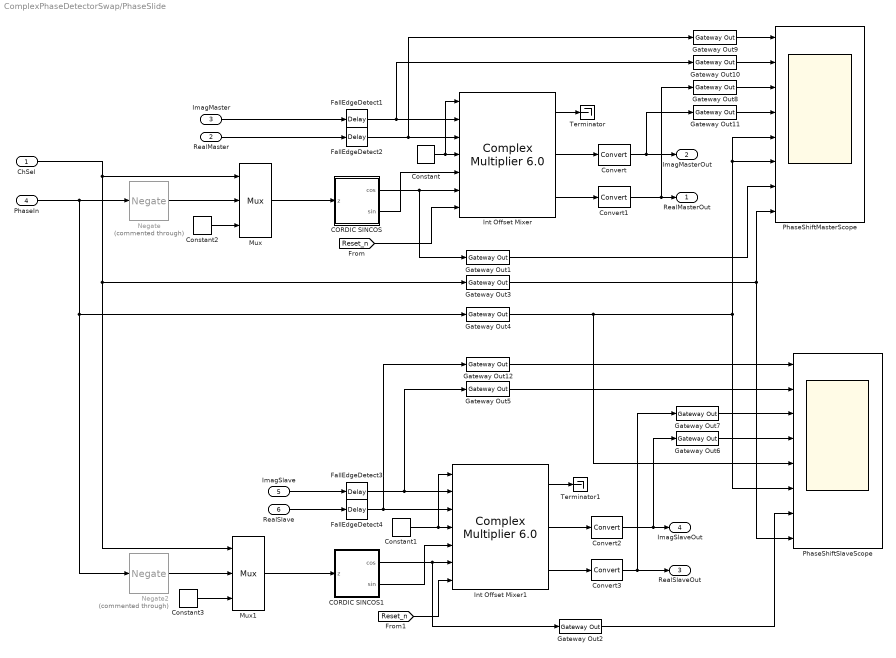
== system ComplexPhaseDetectorSwap/PhaseSlide ==
  ChSel : Inport
  RealMaster : Inport  Port=2
  ImagMaster : Inport  Port=3
  PhaseIn : Inport  Port=4
  ImagSlave : Inport  Port=5
  RealSlave : Inport  Port=6
  CORDIC SINCOS : Subsystem  mask(Xilinx CORDIC SINCOS){stages=17, pe_nbits=21, pe_binpt=17, pipeline_x=ones(1,17), prev_stages=17, pipeline=[1  1  1  1  1  1  1  1  1  1  1  1  1  1  1  1  1]}
      mask prompts: stages "Number of Processing Elements (integer value starting from 1)"; pe_nbits "Input Data Width"; pe_binpt "Input Binary Point Position"; pipeline_x "Latency for each Processing Element [1 0 0 1]"; prev_stages "Previous Number of Stages"; pipeline "Previous Pipeline Values"
      mask help: A parallel implementation, circular rotation mode CORDIC processor for calculating Sine and Cosine of input angle z. The number of iteration stages (and resultant output accuracy) and the processor arithmetic precision are controlled by the mask customization.
      mask init: same as ComplexPhaseDetectorSwap/Bipolar NCO/CORDIC SINCOS
      settings: CopyFcn=set_param(gcb, 'MaskSelfModifiable', 'on', 'LinkStatus', 'none');
      mask Help: eval('');xlDoc('-book','sysgen','-topic','CORDIC_SINCOS');
      mask Display:
      | patch([0 iWidth iWidth 0],[0 0 iHeight iHeight] , bg);
      | patch(logoX,logoY , fg);
      | text(iCx-6,iCy,'z');
      | text(iCx,iCy+4,str);
      | port_label('input',1,'z');
      | port_label('output',1,'cos');
      | port_label('output',2,'sin');
      | plot([0 0 iWidth iWidth 0], [0 iHeight iHeight 0 0]);
  CORDIC SINCOS1 : Subsystem  mask(Xilinx CORDIC SINCOS){stages=17, pe_nbits=21, pe_binpt=17, pipeline_x=ones(1,17), prev_stages=17, pipeline=[1  1  1  1  1  1  1  1  1  1  1  1  1  1  1  1  1]}
      mask prompts: stages "Number of Processing Elements (integer value starting from 1)"; pe_nbits "Input Data Width"; pe_binpt "Input Binary Point Position"; pipeline_x "Latency for each Processing Element [1 0 0 1]"; prev_stages "Previous Number of Stages"; pipeline "Previous Pipeline Values"
      mask help: A parallel implementation, circular rotation mode CORDIC processor for calculating Sine and Cosine of input angle z. The number of iteration stages (and resultant output accuracy) and the processor arithmetic precision are controlled by the mask customization.
      mask init: same as ComplexPhaseDetectorSwap/Bipolar NCO/CORDIC SINCOS
      settings: CopyFcn=set_param(gcb, 'MaskSelfModifiable', 'on', 'LinkStatus', 'none');
      mask Help: eval('');xlDoc('-book','sysgen','-topic','CORDIC_SINCOS');
      mask Display:
      | patch([0 iWidth iWidth 0],[0 0 iHeight iHeight] , bg);
      | patch(logoX,logoY , fg);
      | text(iCx-6,iCy,'z');
      | text(iCx,iCy+4,str);
      | port_label('input',1,'z');
      | port_label('output',1,'cos');
      | port_label('output',2,'sin');
      | plot([0 0 iWidth iWidth 0], [0 iHeight iHeight 0 0]);
  Constant : xbsIndex_r4/Constant  const=1  gui_display_data_type=Boolean  arith_type=Boolean  n_bits=16  bin_pt=14  preci_type=Single  exp_width=8  frac_width=24  explicit_period=on  period=Ts  equ=P=C  opselect=C  inp2=PCIN>>17  opr=+  inp1=P  carry=CIN  dbl_ovrd=off  block_type=constant
  Constant1 : xbsIndex_r4/Constant  const=1  gui_display_data_type=Boolean  arith_type=Boolean  n_bits=16  bin_pt=14  preci_type=Single  exp_width=8  frac_width=24  explicit_period=on  period=Ts  equ=P=C  opselect=C  inp2=PCIN>>17  opr=+  inp1=P  carry=CIN  dbl_ovrd=off  block_type=constant
  Constant2 : xbsIndex_r4/Constant  const=0  gui_display_data_type=Fixed-point  arith_type=Signed (2's comp)  n_bits=16  bin_pt=14  preci_type=Single  exp_width=8  frac_width=24  explicit_period=on  period=Ts  equ=P=C  opselect=C  inp2=PCIN>>17  opr=+  inp1=P  carry=CIN  dbl_ovrd=off  block_type=constant
  Constant3 : xbsIndex_r4/Constant  const=0  gui_display_data_type=Fixed-point  arith_type=Signed (2's comp)  n_bits=16  bin_pt=14  preci_type=Single  exp_width=8  frac_width=24  explicit_period=on  period=Ts  equ=P=C  opselect=C  inp2=PCIN>>17  opr=+  inp1=P  carry=CIN  dbl_ovrd=off  block_type=constant
  Convert{,1..3} (4 alike) : xbsIndex_r4/Convert  gui_display_data_type=Fixed-point  arith_type="Signed  (2's comp)"  n_bits=18  bin_pt=17  float_type=Single  exp_bits=8  fraction_bits=24  quantization=Truncate  overflow=Saturate  en=off  latency=1  pipeline=off  dbl_ovrd=off  block_type=convert
  FallEdgeDetect{1..4} (4 alike) : xbsIndex_r4/Delay  rst=off  infoeditControl=Selection of Reset will increase slice count due to use of real FFs and instead of SRLs  en=off  latency=42  reg_retiming=off  dbl_ovrd=off  block_type=delay
  Gateway Out{1..12} (12 alike) : xbsIndex_r4/Gateway Out  inherit_from_input=off  hdl_port=off  rows=1  columns=1  UseAsDAC=off  DACChannel='1'  interface=None  automatic_assignment=on  address_offset=hex2dec('00')  intf_name=''  intf_description=''  timing_constraint=None  locs_specified=off  LOCs={}  io_standard={}  block_type=gatewayout
  Int Offset Mixer : xbsIndex_r4/Complex Multiplier 6.0   hasatlast=off  hasatuser=off  atuserwidth=1  hasbtlast=off  hasbtuser=off  btuserwidth=1  multtype=Use_Mults  optimizegoal=Resources  flowcontrol=NonBlocking  outputwidth=20  roundmode=Truncate  hasctrltlast=off  hasctrltuser=off  ctrltuserwidth=1  outtlastbehv=Null  latencyconfig=Manual  minimumlatency=3  aclken=off  aresetn=on  trim_axipin_name=on  simulation_type=hybrid_sim  simulation_model=sysgen:cmpy_v6_0  data_path_portlist={ 's_axis_a_tdata_real', 's_axis_a_tdata_imag', 's_axis_b_tdata_real', 's_axis_b_tdata_imag', 's_axis_ctrl_tdata_rounding_bit', 'm_axis_dout_tdata_real', 'm_axis_dout_tdata_imag' }  aportwidth=63  bportwidth=63  ip_name=Complex Multiplier  ip_version=6.0  dsptool_ready=true  ipcore_usecache=true  ipcore_useipmodelcache=true  ipcore_verbose=false  ipcore_latency_parameter='minimumlatency'  wrapper_available=true  port_translation_map={ 'aclken' => 'en', 'aresetn' => 'rst'}  block_type=cmpy_v6_0
  Int Offset Mixer1 : xbsIndex_r4/Complex Multiplier 6.0   hasatlast=off  hasatuser=off  atuserwidth=1  hasbtlast=off  hasbtuser=off  btuserwidth=1  multtype=Use_Mults  optimizegoal=Resources  flowcontrol=NonBlocking  outputwidth=20  roundmode=Truncate  hasctrltlast=off  hasctrltuser=off  ctrltuserwidth=1  outtlastbehv=Null  latencyconfig=Manual  minimumlatency=3  aclken=off  aresetn=on  trim_axipin_name=on  simulation_type=hybrid_sim  simulation_model=sysgen:cmpy_v6_0  data_path_portlist={ 's_axis_a_tdata_real', 's_axis_a_tdata_imag', 's_axis_b_tdata_real', 's_axis_b_tdata_imag', 's_axis_ctrl_tdata_rounding_bit', 'm_axis_dout_tdata_real', 'm_axis_dout_tdata_imag' }  aportwidth=63  bportwidth=63  ip_name=Complex Multiplier  ip_version=6.0  dsptool_ready=true  ipcore_usecache=true  ipcore_useipmodelcache=true  ipcore_verbose=false  ipcore_latency_parameter='minimumlatency'  wrapper_available=true  port_translation_map={ 'aclken' => 'en', 'aresetn' => 'rst'}  block_type=cmpy_v6_0
  Mux : xbsIndex_r4/Mux  inputs=2  en=off  latency=1  precision=Full  arith_type=Unsigned  n_bits=16  bin_pt=14  quantization=Truncate  overflow=Wrap  dbl_ovrd=off  block_type=mux
  Mux1 : xbsIndex_r4/Mux  inputs=2  en=off  latency=1  precision=Full  arith_type=Unsigned  n_bits=16  bin_pt=14  quantization=Truncate  overflow=Wrap  dbl_ovrd=off  block_type=mux
  Negate : xbsIndex_r4/Negate  Commented=through  precision=User Defined  arith_type="Signed  (2's comp)"  n_bits=21  bin_pt=17  quantization=Truncate  overflow=Saturate  en=off  latency=1  dbl_ovrd=off  block_type=negate
  Negate2 : xbsIndex_r4/Negate  Commented=through  precision=User Defined  arith_type="Signed  (2's comp)"  n_bits=21  bin_pt=17  quantization=Truncate  overflow=Saturate  en=off  latency=1  dbl_ovrd=off  block_type=negate
  PhaseShiftMasterScope : Scope  NumInputPorts=8
  PhaseShiftSlaveScope : Scope  NumInputPorts=8
  Terminator : Terminator
  Terminator1 : Terminator
  RealMasterOut : Outport
  ImagMasterOut : Outport  Port=2
  RealSlaveOut : Outport  Port=3
  ImagSlaveOut : Outport  Port=4
  wires:
  Constant/1 -> Int Offset Mixer/1, Int Offset Mixer/4
  CORDIC SINCOS/2(sin) -> Int Offset Mixer/5
  Int Offset Mixer/1 -> Terminator/1
  Convert1/1 -> Gateway Out8/1, RealMasterOut/1
  RealMaster/1 -> FallEdgeDetect2/1
  Convert/1 -> Gateway Out11/1, ImagMasterOut/1
  CORDIC SINCOS/1(cos) -> Gateway Out1/1, Int Offset Mixer/6
  Gateway Out1/1 -> PhaseShiftMasterScope/7
  Int Offset Mixer/3 -> Convert1/1
  Int Offset Mixer/2 -> Convert/1
  Gateway Out3/1 -> PhaseShiftMasterScope/8, PhaseShiftSlaveScope/8
  ImagSlave/1 -> FallEdgeDetect3/1
  Constant1/1 -> Int Offset Mixer1/1, Int Offset Mixer1/4
  CORDIC SINCOS1/2(sin) -> Int Offset Mixer1/5
  Int Offset Mixer1/1 -> Terminator1/1
  RealSlave/1 -> FallEdgeDetect4/1
  Convert2/1 -> Gateway Out6/1, ImagSlaveOut/1
  CORDIC SINCOS1/1(cos) -> Gateway Out2/1, Int Offset Mixer1/6
  Mux1/1 -> CORDIC SINCOS1/1(z)
  Int Offset Mixer1/3 -> Convert3/1
  Int Offset Mixer1/2 -> Convert2/1
  [Reset_n] -> Int Offset Mixer/7
  Gateway Out9/1 -> PhaseShiftMasterScope/1
  Gateway Out10/1 -> PhaseShiftMasterScope/2
  Gateway Out8/1 -> PhaseShiftMasterScope/3
  Gateway Out11/1 -> PhaseShiftMasterScope/4
  FallEdgeDetect1/1 -> Gateway Out10/1, Int Offset Mixer/2
  FallEdgeDetect2/1 -> Gateway Out9/1, Int Offset Mixer/3
  FallEdgeDetect3/1 -> Gateway Out5/1, Int Offset Mixer1/2
  FallEdgeDetect4/1 -> Gateway Out12/1, Int Offset Mixer1/3
  Gateway Out4/1 -> PhaseShiftSlaveScope/5, PhaseShiftMasterScope/5, PhaseShiftMasterScope/6, PhaseShiftSlaveScope/6
  ImagMaster/1 -> FallEdgeDetect1/1
  Mux/1 -> CORDIC SINCOS/1(z)
  Constant2/1 -> Mux/3
  Negate/1 -> Mux/2
  PhaseIn/1 -> Negate2/1, Gateway Out4/1, Negate/1
  Constant3/1 -> Mux1/3
  Gateway Out12/1 -> PhaseShiftSlaveScope/1
  Gateway Out5/1 -> PhaseShiftSlaveScope/2
  Gateway Out7/1 -> PhaseShiftSlaveScope/3
  Gateway Out6/1 -> PhaseShiftSlaveScope/4
  [Reset_n] -> Int Offset Mixer1/7
  Convert3/1 -> Gateway Out7/1, RealSlaveOut/1
  Gateway Out2/1 -> PhaseShiftSlaveScope/7
  ChSel/1 -> Mux1/1, Gateway Out3/1, Mux/1
  Negate2/1 -> Mux1/2

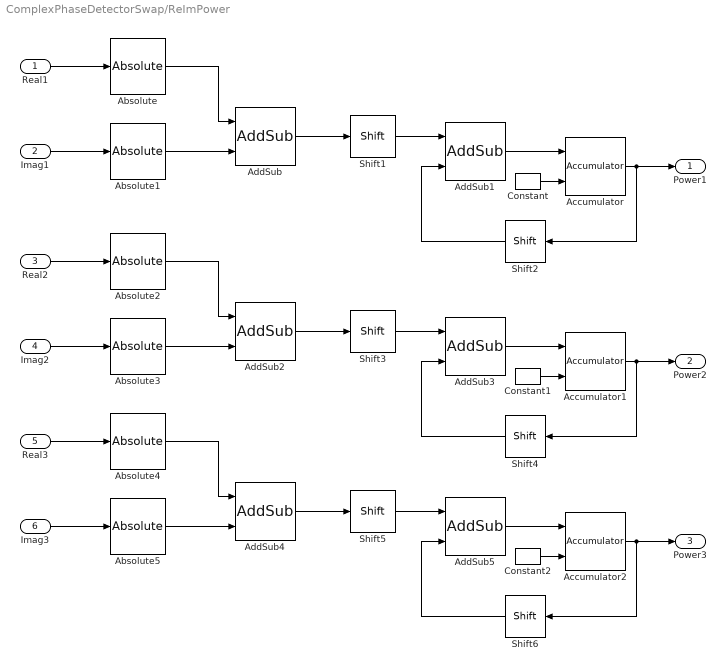
== system ComplexPhaseDetectorSwap/ReImPower ==
  Real1 : Inport
  Imag1 : Inport  Port=2
  Real2 : Inport  Port=3
  Imag2 : Inport  Port=4
  Real3 : Inport  Port=5
  Imag3 : Inport  Port=6
  Absolute{,1..5} (6 alike) : xbsIndex_r4/Absolute  precision=Full  arith_type=Unsigned  n_bits=16  bin_pt=14  quantization=Truncate  overflow=Wrap  en=off  latency=0  dbl_ovrd=off  block_type=abs
  Accumulator : xbsIndex_r4/Accumulator  operation=Add  n_bits=21  overflow=Wrap  scale=1  rst=on  hasbypass=off  infoeditControl=reset for floating point data type must be asserted for a minimum of 2 cycles  en=off  latency=1  msb_inp=100  msb=100  lsb=-100  use_behavioral_HDL=on  implementation=Fabric  dbl_ovrd=off  block_type=accum
  Accumulator1 : xbsIndex_r4/Accumulator  operation=Add  n_bits=21  overflow=Wrap  scale=1  rst=on  hasbypass=off  infoeditControl=reset for floating point data type must be asserted for a minimum of 2 cycles  en=off  latency=1  msb_inp=100  msb=100  lsb=-100  use_behavioral_HDL=on  implementation=Fabric  dbl_ovrd=off  block_type=accum
  Accumulator2 : xbsIndex_r4/Accumulator  operation=Add  n_bits=21  overflow=Wrap  scale=1  rst=on  hasbypass=off  infoeditControl=reset for floating point data type must be asserted for a minimum of 2 cycles  en=off  latency=1  msb_inp=100  msb=100  lsb=-100  use_behavioral_HDL=on  implementation=Fabric  dbl_ovrd=off  block_type=accum
  AddSub : xbsIndex_r4/AddSub  mode=Addition  use_carryin=off  use_carryout=off  en=off  latency=1  precision=Full  arith_type=Unsigned  n_bits=16  bin_pt=14  quantization=Truncate  overflow=Wrap  use_behavioral_HDL=off  hw_selection=Fabric  pipelined=off  dbl_ovrd=off  block_type=addsub
  AddSub1 : xbsIndex_r4/AddSub  mode=Subtraction  use_carryin=off  use_carryout=off  en=off  latency=1  precision=Full  arith_type=Unsigned  n_bits=16  bin_pt=14  quantization=Truncate  overflow=Wrap  use_behavioral_HDL=off  hw_selection=Fabric  pipelined=off  dbl_ovrd=off  block_type=addsub
  AddSub2 : xbsIndex_r4/AddSub  mode=Addition  use_carryin=off  use_carryout=off  en=off  latency=1  precision=Full  arith_type=Unsigned  n_bits=16  bin_pt=14  quantization=Truncate  overflow=Wrap  use_behavioral_HDL=off  hw_selection=Fabric  pipelined=off  dbl_ovrd=off  block_type=addsub
  AddSub3 : xbsIndex_r4/AddSub  mode=Subtraction  use_carryin=off  use_carryout=off  en=off  latency=1  precision=Full  arith_type=Unsigned  n_bits=16  bin_pt=14  quantization=Truncate  overflow=Wrap  use_behavioral_HDL=off  hw_selection=Fabric  pipelined=off  dbl_ovrd=off  block_type=addsub
  AddSub4 : xbsIndex_r4/AddSub  mode=Addition  use_carryin=off  use_carryout=off  en=off  latency=1  precision=Full  arith_type=Unsigned  n_bits=16  bin_pt=14  quantization=Truncate  overflow=Wrap  use_behavioral_HDL=off  hw_selection=Fabric  pipelined=off  dbl_ovrd=off  block_type=addsub
  AddSub5 : xbsIndex_r4/AddSub  mode=Subtraction  use_carryin=off  use_carryout=off  en=off  latency=1  precision=Full  arith_type=Unsigned  n_bits=16  bin_pt=14  quantization=Truncate  overflow=Wrap  use_behavioral_HDL=off  hw_selection=Fabric  pipelined=off  dbl_ovrd=off  block_type=addsub
  Constant : xbsIndex_r4/Constant  const=0  gui_display_data_type=Boolean  arith_type=Boolean  n_bits=16  bin_pt=14  preci_type=Single  exp_width=8  frac_width=24  explicit_period=off  period=1  equ=P=C  opselect=C  inp2=PCIN>>17  opr=+  inp1=P  carry=CIN  dbl_ovrd=off  block_type=constant
  Constant1 : xbsIndex_r4/Constant  const=0  gui_display_data_type=Boolean  arith_type=Boolean  n_bits=16  bin_pt=14  preci_type=Single  exp_width=8  frac_width=24  explicit_period=off  period=1  equ=P=C  opselect=C  inp2=PCIN>>17  opr=+  inp1=P  carry=CIN  dbl_ovrd=off  block_type=constant
  Constant2 : xbsIndex_r4/Constant  const=0  gui_display_data_type=Boolean  arith_type=Boolean  n_bits=16  bin_pt=14  preci_type=Single  exp_width=8  frac_width=24  explicit_period=off  period=1  equ=P=C  opselect=C  inp2=PCIN>>17  opr=+  inp1=P  carry=CIN  dbl_ovrd=off  block_type=constant
  Shift{1..6} (6 alike) : xbsIndex_r4/Shift  shift_dir=Right  shift_bits=N  en=off  latency=0  precision=Full  arith_type="Signed  (2's comp)"  n_bits=16  bin_pt=14  quantization=Truncate  overflow=Wrap  dbl_ovrd=off  block_type=shift
  Power1 : Outport
  Power2 : Outport  Port=2
  Power3 : Outport  Port=3
  wires:
  Real1/1 -> Absolute/1
  Imag1/1 -> Absolute1/1
  Accumulator/1 -> Shift2/1, Power1/1
  Absolute/1 -> AddSub/1
  Constant/1 -> Accumulator/2
  Shift2/1 -> AddSub1/2
  Shift1/1 -> AddSub1/1
  Absolute1/1 -> AddSub/2
  AddSub/1 -> Shift1/1
  AddSub1/1 -> Accumulator/1
  Real2/1 -> Absolute2/1
  Imag2/1 -> Absolute3/1
  Accumulator1/1 -> Power2/1, Shift4/1
  Absolute2/1 -> AddSub2/1
  Constant1/1 -> Accumulator1/2
  Shift4/1 -> AddSub3/2
  Shift3/1 -> AddSub3/1
  Absolute3/1 -> AddSub2/2
  AddSub2/1 -> Shift3/1
  AddSub3/1 -> Accumulator1/1
  Real3/1 -> Absolute4/1
  Imag3/1 -> Absolute5/1
  Accumulator2/1 -> Shift6/1, Power3/1
  Absolute4/1 -> AddSub4/1
  Constant2/1 -> Accumulator2/2
  Shift6/1 -> AddSub5/2
  Shift5/1 -> AddSub5/1
  Absolute5/1 -> AddSub4/2
  AddSub4/1 -> Shift5/1
  AddSub5/1 -> Accumulator2/1
